simulink model "Houghline_real_fast_2"  (R2016a)
settings: Solver=FixedStepAuto  StartTime=0.0  StopTime=100  RelTol=1e-3
model workspace (MATLAB code in the model file):
  | %% define
  | imagesize = [480 640];
  | cropsize = [240 640];
  | H_start = 240;
  | W_start = 1;
  | %cropsize = [imagesize(1)-H_start imagesize(2)-W_start];
  | number_local_max = 15;
  | %% molp
  | %erode_constant = strel('square',2);
  | erode_constant = 1;
  | %dilation_constant = [1 1;1 1];
  | dilation_constant = 1;
undefined symbols (not defined in the file): gray, Rec, SDTV
libraries: visionconversions x5, visiontextngfix x5, visionmorphops x3, visiontransforms x3, visionfilter x2, dspvision x1, visionanalysis x1, visionstatistics x1
settings Model: Creator=Yewly  LastModifiedBy=Yewly
settings GRTTargetCC: GeneratePreprocessorConditionals=Use local settings

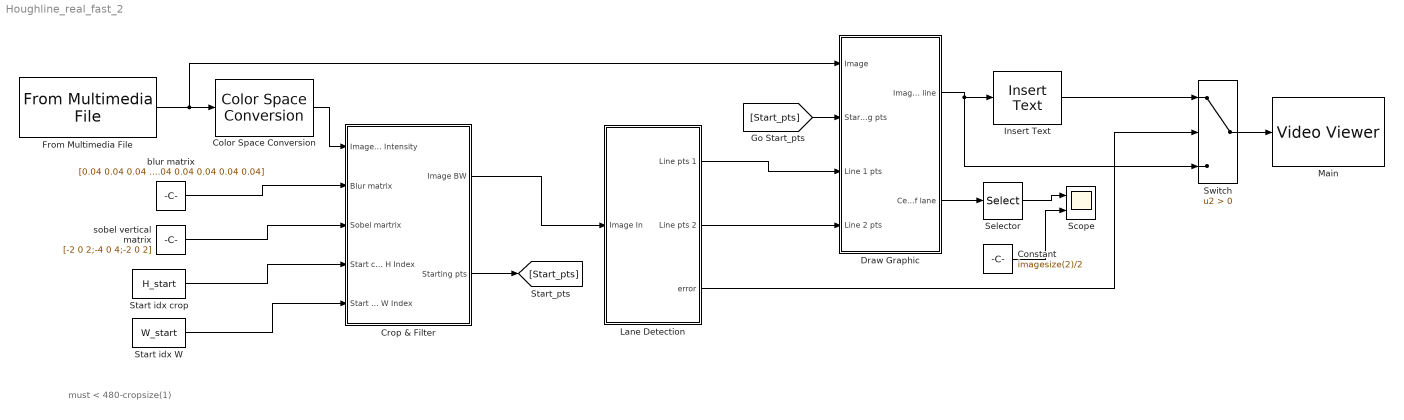
== system Houghline_real_fast_2 ==
  note: must < 480-cropsize(1)
  Color Space Conversion : visionconversions/Color Space  Conversion  conversion=Obsolete  conversionActive=R'G'B' to intensity  wp_str=D65  rec=Rec. 601 (SDTV)  sys=1125/60/2:1  imagePorts=One multidimensional signal
  Constant : Constant  Value=imagesize(2)/2
  Crop & Filter : Subsystem
  Draw Graphic : Subsystem
  From Multimedia File : dspvision/From Multimedia File  inputFilename=lane2.mp4  loop=on  numPlays=inf  outputStreams=Video only  videoDataType=single  audioDataType=int16  inheritSampleTime=on  userDefinedSampleTime=1/5  noAudioOutput=off  isIntensityVideo=off  fourcc=RGB  colorVideoFormat=One multidimensional signal  outputEOF=off  dataOrg=Column-major  audioFrameSize=1024  computeAudioFrameSize=off  outSamplingMode=Sample based
  Insert Text : visiontextngfix/Insert Text  inputType=Obsolete  theText='ERROR'  getTextLocFrom=Specify via dialog  textLoc=[20 20]  getTextColorFrom=Specify via dialog  textColor=[255 0 0]  getTextIntensityFrom=Specify via dialog  textIntensity=0  getTextOpacityFrom=Specify via dialog  textOpacity=1.0  dummyVar2=0  dummyVar3=0  dummyVar4=0  imagePorts=One multidimensional signal  isInputTransposed=off  fontFace=LucidaSansRegular  dummyVar1=0  blockFontSize=32  antiAliased=on
  Lane Detection : Subsystem
  Main : VideoViewer  colormapValue=gray(256)  FigPos=[-3 606.8 689.6 501.6]
  Scope : Scope  NumInputPorts=2
  Selector : Selector  NumberOfDimensions=2  InputPortWidth=3  IndexOptions=Index vector (dialog),Index vector (dialog)  Indices=1,1  OutputSizes=1,1
  Start idx W : Constant  Value=W_start  OutDataTypeStr=double
  Start idx crop : Constant  Value=H_start  OutDataTypeStr=double
  Switch : Switch  Criteria=u2 > Threshold
  blur matrix : Constant  Value=[0.04 0.04 0.04 0.04 0.04;0.04 0.04 0.04 0.04 0.04;0.04 0.04 0.04 0.04 0.04;0.04 0.04 0.04 0.04 0.04;0.04 0.04 0.04 0.04 0.04]  OutDataTypeStr=double
  sobel vertical matrix : Constant  Value=[-2 0 2;-4 0 4;-2 0 2]  OutDataTypeStr=double
  wires:
  Switch/1 -> Main/1
  Lane Detection/3(error) -> Switch/2
  Insert Text/1 -> Switch/1
  Crop & Filter/1(Image BW) -> Lane Detection/1(Image In)
  Color Space Conversion/1 -> Crop & Filter/1(Image Intensity)
  blur matrix/1 -> Crop & Filter/2(Blur matrix)
  sobel vertical matrix/1 -> Crop & Filter/3(Sobel martrix)
  Start idx crop/1 -> Crop & Filter/4(Start crop H Index)
  Crop & Filter/2(Starting pts) -> [Start_pts]
  [Start_pts] -> Draw Graphic/2(Starting pts)
  From Multimedia File/1 -> Draw Graphic/1("Image "), Color Space Conversion/1
  Lane Detection/1(Line pts 1) -> Draw Graphic/3(Line 1 pts)
  Lane Detection/2(Line pts 2) -> Draw Graphic/4(Line 2 pts)
  Draw Graphic/1("Image draw line ") -> Switch/3, Insert Text/1
  Draw Graphic/2(Center point of lane) -> Selector/1
  Selector/1 -> Scope/1
  Constant/1 -> Scope/2
  Start idx W/1 -> Crop & Filter/5(Start crop W Index)

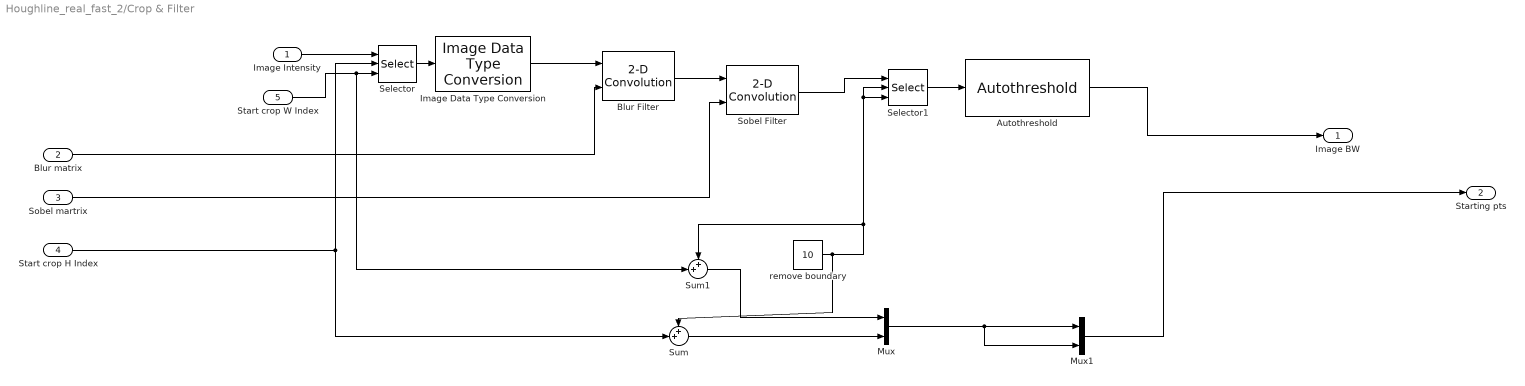
== system Houghline_real_fast_2/Crop & Filter ==
  Image Intensity : Inport
  Blur matrix : Inport  Port=2
  Sobel martrix : Inport  Port=3
  Start crop H Index : Inport  Port=4
  Start crop W Index : Inport  Port=5
  Autothreshold : visionconversions/Autothreshold  operator=>  threshOut=off  effMetricOut=off  userDefinedRange=off  umin=0  umax=255  outOfRngOpt=Warn and saturate  scaleThreshold=off  scaleFactor=1  P1Mode=Specify word length  P1WordLength=32  P1FracLength=30  P2Mode=Specify word length  P2WordLength=32  P2FracLength=22  P3Mode=Specify word length  P3WordLength=32  P3FracLength=14  P4Mode=Binary point scaling  P4WordLength=32  P4FracLength=15  Q1Mode=Specify word length  Q1WordLength=32  Q1FracLength=16  EMMode=Specify word length  EMWordLength=16  EMFracLength=14  roundingMode=Floor  overflowMode=off
  Blur Filter : visionfilter/2-D Convolution  outSize=Full  normalize=off  outputMode=Binary point scaling  outputWordLength=32  outputFracLength=12  prodOutputMode=Binary point scaling  prodOutputWordLength=32  prodOutputFracLength=10  roundingMode=Floor  overflowMode=off
  Image Data Type Conversion : visionconversions/Image Data Type Conversion  outDT=double  isSigned=on  wordLen=16  numFracBits=0
  Mux : Mux  Inputs=2
  Mux1 : Mux  Inputs=2
  Selector : Selector  NumberOfDimensions=2  InputPortWidth=3  IndexOptions=Starting index (port),Starting index (port)  Indices=220,1  OutputSizes=cropsize(1),cropsize(2)
  Selector1 : Selector  NumberOfDimensions=2  InputPortWidth=3  IndexOptions=Starting index (port),Starting index (port)  Indices=10,10  OutputSizes=cropsize(1)-10,cropsize(2)-10
  Sobel Filter : visionfilter/2-D Convolution  outSize=Full  normalize=off  outputMode=Binary point scaling  outputWordLength=32  outputFracLength=12  prodOutputMode=Binary point scaling  prodOutputWordLength=32  prodOutputFracLength=10  roundingMode=Floor  overflowMode=off
  Sum : Sum  Inputs=++|
  Sum1 : Sum  Inputs=++|
  remove boundary : Constant  Value=10  OutDataTypeStr=double
  Image BW : Outport
  Starting pts : Outport  Port=2
  wires:
  Selector/1 -> Image Data Type Conversion/1
  Mux/1 -> Mux1/2, Mux1/1
  Mux1/1 -> Starting pts/1
  Sum/1 -> Mux/2
  Start crop H Index/1 -> Selector/2, Sum/2
  Sobel martrix/1 -> Sobel Filter/2
  Blur matrix/1 -> Blur Filter/2
  Blur Filter/1 -> Sobel Filter/1
  Sobel Filter/1 -> Selector1/1
  Selector1/1 -> Autothreshold/1
  Image Data Type Conversion/1 -> Blur Filter/1
  Image Intensity/1 -> Selector/1
  remove boundary/1 -> Sum1/1, Selector1/3, Selector1/2, Sum/1
  Autothreshold/1 -> Image BW/1
  Start crop W Index/1 -> Sum1/2, Selector/3
  Sum1/1 -> Mux/1

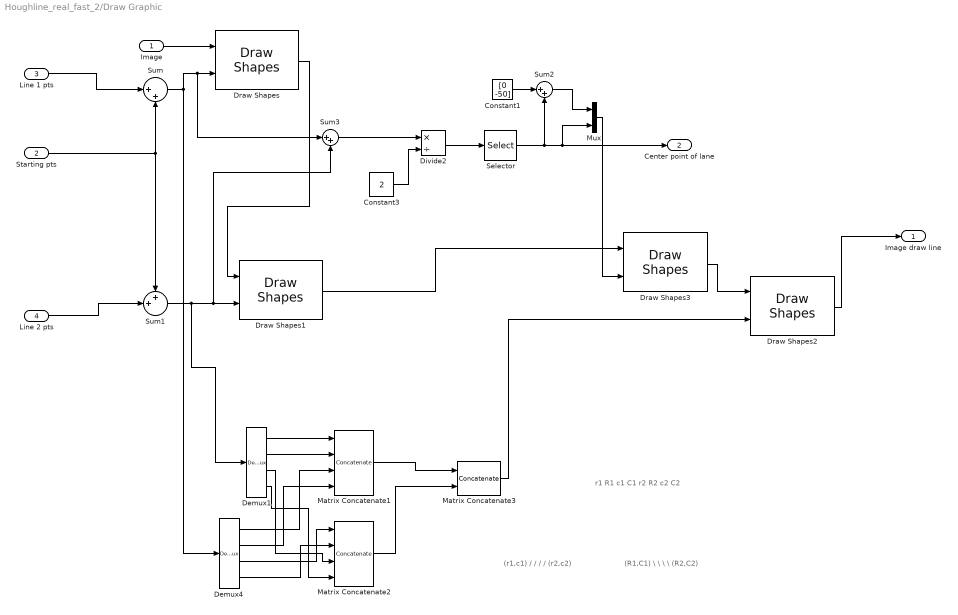
== system Houghline_real_fast_2/Draw Graphic ==
  note: r1   R1
      | c1   C1
      | r2   R2
      | c2   C2
  note: (r1,c1)
      |                        /
      |                    /
      |               /
      |          /
      | (r2,c2)
  note: (R1,C1)
      |  \
      |        \
      |            \
      |                  \
      |                        (R2,C2)
  "Image " : Inport
  Starting pts : Inport  Port=2
  Line 1 pts : Inport  Port=3
  Line 2 pts : Inport  Port=4
  Constant1 : Constant  Value=[0 -50]
  Constant3 : Constant  Value=2
  Demux1 : Demux
  Demux4 : Demux
  Divide2 : Product  Inputs=*/
  Draw Shapes : visiontextngfix/Draw Shapes  shape=Lines  fill=off  lineWidth=4  fillClrSource=Specify via dialog  display=User-specified value  intensity=200  color=[0 255 0]  opacity=0.6  viewport=Entire image  antialiasing=off  inType=Obsolete  imagePorts=One multidimensional signal  prodOutputMode=Binary point scaling  prodOutputWordLength=32  prodOutputFracLength=14  memoryMode=Specify word length  memoryWordLength=16  memoryFracLength=14  roundingMode=Floor  overflowMode=off
  Draw Shapes1 : visiontextngfix/Draw Shapes  shape=Lines  fill=off  lineWidth=4  fillClrSource=Specify via dialog  display=User-specified value  intensity=200  color=[0 0 255]  opacity=0.6  viewport=Entire image  antialiasing=off  inType=Obsolete  imagePorts=One multidimensional signal  prodOutputMode=Binary point scaling  prodOutputWordLength=32  prodOutputFracLength=14  memoryMode=Specify word length  memoryWordLength=16  memoryFracLength=14  roundingMode=Floor  overflowMode=off
  Draw Shapes2 : visiontextngfix/Draw Shapes  shape=Polygons  fill=on  lineWidth=1  fillClrSource=Specify via dialog  display=User-specified value  intensity=200  color=[1 0 1]  opacity=0.2  viewport=Entire image  antialiasing=on  inType=Obsolete  imagePorts=One multidimensional signal  prodOutputMode=Binary point scaling  prodOutputWordLength=32  prodOutputFracLength=14  memoryMode=Specify word length  memoryWordLength=16  memoryFracLength=14  roundingMode=Floor  overflowMode=off
  Draw Shapes3 : visiontextngfix/Draw Shapes  shape=Lines  fill=off  lineWidth=4  fillClrSource=Specify via dialog  display=User-specified value  intensity=200  color=[127 127 0]  opacity=0.6  viewport=Entire image  antialiasing=off  inType=Obsolete  imagePorts=One multidimensional signal  prodOutputMode=Binary point scaling  prodOutputWordLength=32  prodOutputFracLength=14  memoryMode=Specify word length  memoryWordLength=16  memoryFracLength=14  roundingMode=Floor  overflowMode=off
  Matrix Concatenate1 : Concatenate  NumInputs=4  Mode=Multidimensional array  ConcatenateDimension=2
  Matrix Concatenate2 : Concatenate  NumInputs=4  Mode=Multidimensional array  ConcatenateDimension=2
  Matrix Concatenate3 : Concatenate  Mode=Multidimensional array  ConcatenateDimension=2
  Mux : Mux  Inputs=2
  Selector : Selector  NumberOfDimensions=2  InputPortWidth=3  IndexOptions=Index vector (dialog),Index vector (dialog)  Indices=1,[3 4]  OutputSizes=1,1
  Sum : Sum  Inputs=|++
  Sum1 : Sum  Inputs=++|
  Sum2 : Sum  Inputs=|++
  Sum3 : Sum  Inputs=|++
  "Image draw line " : Outport
  Center point of lane : Outport  Port=2
  wires:
  Sum/1 -> Sum3/1, Draw Shapes/2, Demux4/1
  Draw Shapes2/1 -> "Image draw line "/1
  Sum1/1 -> Demux1/1, Draw Shapes1/2, Sum3/2
  "Image "/1 -> Draw Shapes/1
  Line 1 pts/1 -> Sum/1
  Line 2 pts/1 -> Sum1/2
  Starting pts/1 -> Sum/2, Sum1/1
  Draw Shapes/1 -> Draw Shapes1/1
  Demux1/1 -> Matrix Concatenate1/1
  Demux4/3 -> Matrix Concatenate2/1
  Demux1/3 -> Matrix Concatenate2/3
  Demux1/2 -> Matrix Concatenate1/2
  Demux4/1 -> Matrix Concatenate1/3
  Matrix Concatenate3/1 -> Draw Shapes2/2
  Matrix Concatenate2/1 -> Matrix Concatenate3/2
  Matrix Concatenate1/1 -> Matrix Concatenate3/1
  Demux4/2 -> Matrix Concatenate1/4
  Demux4/4 -> Matrix Concatenate2/2
  Demux1/4 -> Matrix Concatenate2/4
  Sum3/1 -> Divide2/1
  Constant3/1 -> Divide2/2
  Divide2/1 -> Selector/1
  Draw Shapes1/1 -> Draw Shapes3/1
  Draw Shapes3/1 -> Draw Shapes2/1
  Selector/1 -> Sum2/2, Center point of lane/1, Mux/2
  Mux/1 -> Draw Shapes3/2
  Constant1/1 -> Sum2/1
  Sum2/1 -> Mux/1

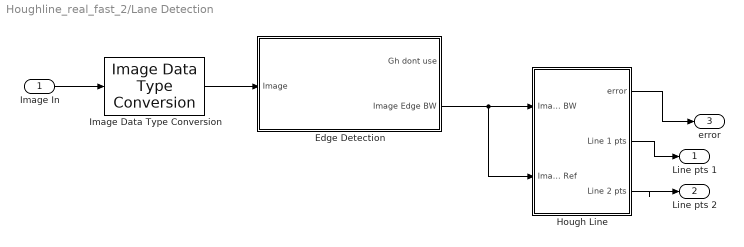
== system Houghline_real_fast_2/Lane Detection ==
  Image In : Inport
  Edge Detection : Subsystem
  Hough Line : Subsystem
  Image Data Type Conversion : visionconversions/Image Data Type Conversion  outDT=double  isSigned=on  wordLen=16  numFracBits=0
  Line pts 1 : Outport
  Line pts 2 : Outport  Port=2
  error : Outport  Port=3
  wires:
  Image Data Type Conversion/1 -> Edge Detection/1("Image ")
  Image In/1 -> Image Data Type Conversion/1
  Hough Line/1(error) -> error/1
  Edge Detection/2(Image Edge BW) -> Hough Line/2(Image Ref), Hough Line/1(Image BW)
  Hough Line/2(Line 1 pts) -> Line pts 1/1
  Hough Line/3(Line 2 pts) -> Line pts 2/1

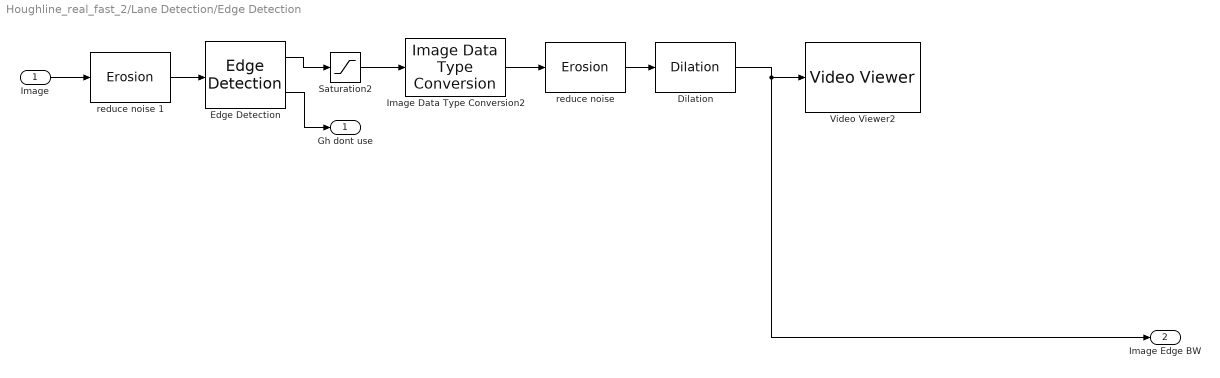
== system Houghline_real_fast_2/Lane Detection/Edge Detection ==
  "Image " : Inport
  Dilation : visionmorphops/Dilation  nhoodsrc=Specify via dialog  strel=dilation_constant
  Edge Detection : visionanalysis/Edge Detection  method=Sobel  outputType=Gradient components  userDefinedThreshold=on  thresholdSource=Specify via dialog  threshold=1  thresholdTuning=1  edgeThinning=on  threshold_canny=[0.25 0.60]  autoPercent=70  sigma=1  prodOutputMode=Binary point scaling  prodOutputWordLength=32  prodOutputFracLength=8  roundingMode=Floor  overflowMode=off
  Image Data Type Conversion2 : visionconversions/Image Data Type Conversion  outDT=boolean  isSigned=on  wordLen=16  numFracBits=0
  Saturation2 : Saturate  UpperLimit=1  LowerLimit=0
  Video Viewer2 : VideoViewer  colormapValue=gray(256)  FigPos=[-28.6 826 690.4 184]
  "reduce noise " : visionmorphops/Erosion  nhoodsrc=Specify via dialog  strel=erode_constant
  reduce noise 1 : visionmorphops/Erosion  nhoodsrc=Specify via dialog  strel=erode_constant
  Gh dont use : Outport
  Image Edge BW : Outport  Port=2
  wires:
  Edge Detection/1 -> Saturation2/1
  "reduce noise "/1 -> Dilation/1
  Saturation2/1 -> Image Data Type Conversion2/1
  Image Data Type Conversion2/1 -> "reduce noise "/1
  reduce noise 1/1 -> Edge Detection/1
  Edge Detection/2 -> Gh dont use/1
  "Image "/1 -> reduce noise 1/1
  Dilation/1 -> Image Edge BW/1, Video Viewer2/1

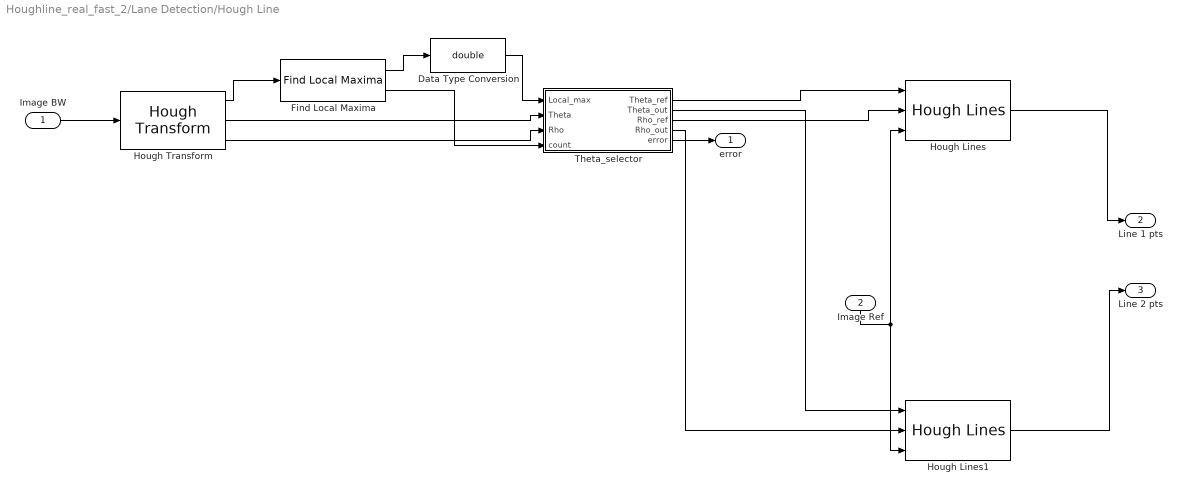
== system Houghline_real_fast_2/Lane Detection/Hough Line ==
  Image BW : Inport
  Image Ref : Inport  Port=2
  Data Type Conversion : DataTypeConversion  OutDataTypeStr=double
  Find Local Maxima : visionstatistics/Find Local Maxima  num_peaks=number_local_max  nhood_size=[5 7]  src_thresh=Obsolete9b  src_thresh_inuse=Specify via dialog  threshold=10  inputIsHough=off  dt_peak=uint32  isOutVarDim=off  dt_count=uint32
  Hough Lines : visiontransforms/Hough Lines  sineCompMethod=Trigonometric function  thetaRes=pi/180  firstCoeffMode=Specify word length  firstCoeffWordLength=16  firstCoeffFracLength=15  prodOutputMode=Binary point scaling  prodOutputWordLength=32  prodOutputFracLength=16  roundingMode=Nearest  overflowMode=on
  Hough Lines1 : visiontransforms/Hough Lines  sineCompMethod=Trigonometric function  thetaRes=pi/180  firstCoeffMode=Specify word length  firstCoeffWordLength=16  firstCoeffFracLength=15  prodOutputMode=Binary point scaling  prodOutputWordLength=32  prodOutputFracLength=16  roundingMode=Nearest  overflowMode=on
  Hough Transform : visiontransforms/Hough Transform  theta_res=pi/360  rho_res=1  out_theta_rho=on  outdtmode=double  firstCoeffMode=Binary point scaling  firstCoeffWordLength=16  firstCoeffFracLength=14  secondCoeffMode=Binary point scaling  secondCoeffWordLength=32  secondCoeffFracLength=16  outputMode=Binary point scaling  outputWordLength=16  outputFracLength=0  accumMode=Binary point scaling  accumWordLength=32  accumFracLength=20  prodOutputMode=Binary point scaling  prodOutputWordLength=32  prodOutputFracLength=20  memoryMode=Binary point scaling  memoryWordLength=32  memoryFracLength=16  roundingMode=Nearest  overflowMode=on
  Theta_selector : MATLAB Function  TreatAsAtomicUnit=on
  error : Outport
  Line 1 pts : Outport  Port=2
  Line 2 pts : Outport  Port=3
  wires:
  Find Local Maxima/2 -> Theta_selector/4(count)
  Image Ref/1 -> Hough Lines/3, Hough Lines1/3
  Image BW/1 -> Hough Transform/1
  Theta_selector/1(Theta_ref) -> Hough Lines/1
  Find Local Maxima/1 -> Data Type Conversion/1
  Theta_selector/4(Rho_out) -> Hough Lines1/2
  Data Type Conversion/1 -> Theta_selector/1(Local_max)
  Theta_selector/5(error) -> error/1
  Hough Transform/2 -> Theta_selector/2(Theta)
  Hough Transform/3 -> Theta_selector/3(Rho)
  Theta_selector/3(Rho_ref) -> Hough Lines/2
  Theta_selector/2(Theta_out) -> Hough Lines1/1
  Hough Transform/1 -> Find Local Maxima/1
  Hough Lines/1 -> Line 1 pts/1
  Hough Lines1/1 -> Line 2 pts/1

== matlab function Houghline_real_fast_2/Lane Detection/Hough Line/Theta_selector ==
  data: Theta_ref output; Theta_out output; Rho_ref output; Local_max input; Theta input; Rho input; Rho_out output; error output; count input
function [Theta_ref,Theta_out,Rho_ref,Rho_out,error] = Theta_selector(Local_max,Theta,Rho,count)
[H,W] = size(Local_max);
error = 0;
%%
if count > 1
for x = 1:H
    if Theta(Local_max(x,1)) > 0
        Theta_ref = Theta(Local_max(x,1));
        Rho_ref = Rho(Local_max(x,2));
        break;
    else
    Theta_ref=Theta(Local_max(x,1));
    Rho_ref = Rho(Local_max(x,2));
    end
end

for x = 1:H
    if Theta(Local_max(x,1)) < 0
        Theta_out = Theta(Local_max(x,1));
        Rho_out = Rho(Local_max(x,2));
        break;
    else
    Theta_out=Theta(Local_max(x,1));
    Rho_out = Rho(Local_max(x,2));
    end
end
%% error

if Theta_out > 1 | Theta_ref > 1
        error = 1;
end
if (Theta_out > 0 && Theta_ref > 0) | (Theta_out < 0 && Theta_ref < 0)
        error = 1;
end
else
    Theta_ref=Theta(Local_max(1,1));
    Rho_ref = Rho(Local_max(1,2));
    Theta_out=Theta(Local_max(1,1));
    Rho_out = Rho(Local_max(1,2));
end
